simulink model "antiwindup"  (Simulink 4.00)
settings: Solver=ode45  StartTime=0.0  StopTime=2  MaxStep=0.001  RelTol=1e-3
settings Model: LastModifiedBy=Gui

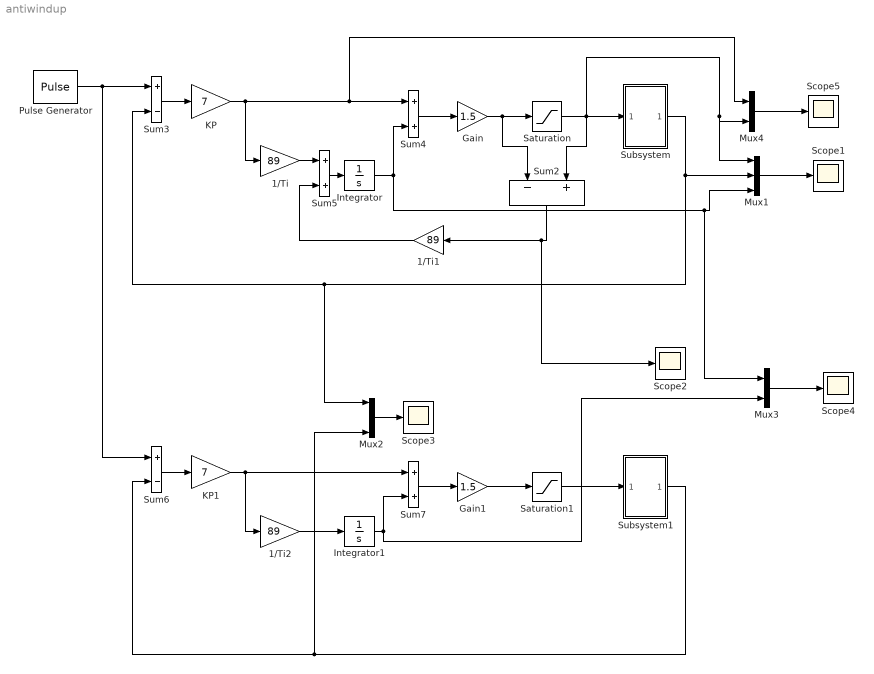
== system antiwindup ==
  1/Ti : Gain  Gain=89  Multiplication=Element-wise(K.*u)  SaturateOnIntegerOverflow=on
  1/Ti1 : Gain  Orientation=left  Gain=89  Multiplication=Element-wise(K.*u)  SaturateOnIntegerOverflow=on
  1/Ti2 : Gain  Gain=89  Multiplication=Element-wise(K.*u)  SaturateOnIntegerOverflow=on
  Gain : Gain  Gain=1.5  Multiplication=Element-wise(K.*u)  SaturateOnIntegerOverflow=on
  Gain1 : Gain  Gain=1.5  Multiplication=Element-wise(K.*u)  SaturateOnIntegerOverflow=on
  Integrator : Integrator  ExternalReset=none  InitialConditionSource=internal  InitialCondition=0  LimitOutput=off  UpperSaturationLimit=inf  LowerSaturationLimit=-inf  ShowSaturationPort=off  ShowStatePort=off  AbsoluteTolerance=auto
  Integrator1 : Integrator  ExternalReset=none  InitialConditionSource=internal  InitialCondition=0  LimitOutput=off  UpperSaturationLimit=inf  LowerSaturationLimit=-inf  ShowSaturationPort=off  ShowStatePort=off  AbsoluteTolerance=auto
  KP : Gain  Gain=7  Multiplication=Element-wise(K.*u)  SaturateOnIntegerOverflow=on
  KP1 : Gain  Gain=7  Multiplication=Element-wise(K.*u)  SaturateOnIntegerOverflow=on
  Mux1 : Mux  Inputs=3
  Mux2 : Mux  Inputs=3
  Mux3 : Mux  Inputs=2
  Mux4 : Mux  Inputs=2
  Pulse Generator : DiscretePulseGenerator  PulseType=Time-based  Amplitude=2  Period=1/5  PulseWidth=50  PhaseDelay=0  SampleTime=1
  Saturation : Saturate  UpperLimit=13.5  LowerLimit=-13.99  LinearizeAsGain=on
  Saturation1 : Saturate  UpperLimit=13.5  LowerLimit=-13.99  LinearizeAsGain=on
  Scope{1..5} (5 alike) : Scope
      Scope1 settings: TimeRange=0.05  YMin=0.2  YMax=1.2  SaveToWorkspace=off  MaxDataPoints=5000
      Scope2 settings: TimeRange=0.05  YMin=-15  YMax=3  SaveToWorkspace=off  SaveName=ScopeData2  MaxDataPoints=5000
      Scope3 settings: TimeRange=0.05  YMin=0.2  YMax=2  SaveToWorkspace=off  SaveName=ScopeData3  MaxDataPoints=5000
      Scope4 settings: TimeRange=0.05  YMin=13.5  YMax=13.5  SaveToWorkspace=off  SaveName=ScopeData4  MaxDataPoints=5000
      Scope5 settings: TimeRange=0.05  YMin=0.2  YMax=1.2  SaveToWorkspace=off  SaveName=ScopeData5  MaxDataPoints=5000
  Subsystem : Subsystem
      settings: RTWFcnNameOpts=Auto  RTWFileNameOpts=Auto
  Subsystem1 : Subsystem
      settings: RTWFcnNameOpts=Auto  RTWFileNameOpts=Auto
  Sum2 : Sum  Orientation=down  Inputs=-+  SaturateOnIntegerOverflow=on
  Sum3 : Sum  Inputs=+-  SaturateOnIntegerOverflow=on
  Sum4 : Sum  Inputs=++  SaturateOnIntegerOverflow=on
  Sum5 : Sum  Inputs=++  SaturateOnIntegerOverflow=on
  Sum6 : Sum  Inputs=+-  SaturateOnIntegerOverflow=on
  Sum7 : Sum  Inputs=++  SaturateOnIntegerOverflow=on
  wires:
  Sum3/1 -> KP/1
  KP/1 -> 1/Ti/1, Sum4/1, Mux4/1
  Gain/1 -> Saturation/1, Sum2/1
  Saturation/1 -> Sum2/2, Mux1/1, Mux4/2, Subsystem/1(In1)
  Sum4/1 -> Gain/1
  1/Ti/1 -> Sum5/1
  Sum5/1 -> Integrator/1
  Integrator/1 -> Sum4/2, Mux1/3, Mux3/1
  Sum2/1 -> 1/Ti1/1, Scope2/1
  1/Ti1/1 -> Sum5/2
  Subsystem/1(Out1) -> Mux1/2, Sum3/2, Mux2/1
  Mux1/1 -> Scope1/1
  Mux2/1 -> Scope3/1
  Sum6/1 -> KP1/1
  KP1/1 -> Sum7/1, 1/Ti2/1
  Gain1/1 -> Saturation1/1
  Saturation1/1 -> Subsystem1/1(In1)
  Sum7/1 -> Gain1/1
  1/Ti2/1 -> Integrator1/1
  Subsystem1/1(Out1) -> Sum6/2, Mux2/3
  Integrator1/1 -> Sum7/2, Mux3/2
  Mux3/1 -> Scope4/1
  Pulse Generator/1 -> Sum3/1, Sum6/1
  Mux4/1 -> Scope5/1

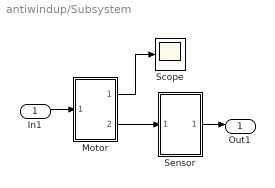
== system antiwindup/Subsystem ==
  In1 : Inport  Port=1  LatchInput=off
  Motor : Subsystem
      settings: RTWFcnNameOpts=Auto  RTWFileNameOpts=Auto
  Scope : Scope
      settings: TimeRange=auto  YMin=-5  YMax=5  SaveToWorkspace=off  SaveName=ScopeData  MaxDataPoints=5000
  Sensor : Subsystem
      settings: RTWFcnNameOpts=Auto  RTWFileNameOpts=Auto
  Out1 : Outport  Port=1
  wires:
  Motor/1(Out1) -> Scope/1
  Motor/2(Out2) -> Sensor/1(In1)
  In1/1 -> Motor/1(In1)
  Sensor/1(Out1) -> Out1/1

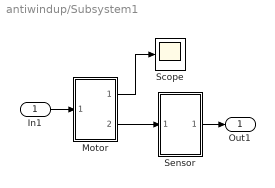
== system antiwindup/Subsystem1 ==
  In1 : Inport  Port=1  LatchInput=off
  Motor : Subsystem
      settings: RTWFcnNameOpts=Auto  RTWFileNameOpts=Auto
  Scope : Scope
      settings: TimeRange=auto  YMin=-5  YMax=5  SaveToWorkspace=off  SaveName=ScopeData  MaxDataPoints=5000
  Sensor : Subsystem
      settings: RTWFcnNameOpts=Auto  RTWFileNameOpts=Auto
  Out1 : Outport  Port=1
  wires:
  Motor/1(Out1) -> Scope/1
  Motor/2(Out2) -> Sensor/1(In1)
  In1/1 -> Motor/1(In1)
  Sensor/1(Out1) -> Out1/1

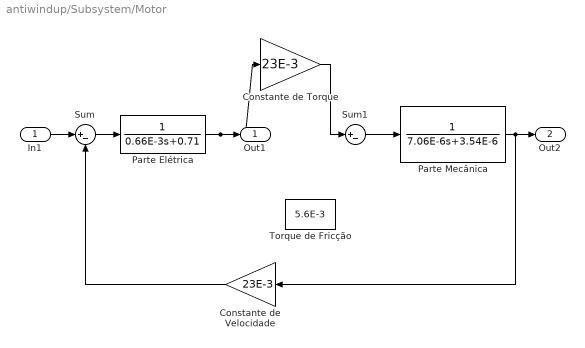
== system antiwindup/Subsystem/Motor ==
  In1 : Inport  Port=1  LatchInput=off
  Constante de Torque : Gain  Gain=23E-3  Multiplication=Element-wise(K.*u)  SaturateOnIntegerOverflow=on
  Constante de Velocidade : Gain  Orientation=left  Gain=23E-3  Multiplication=Element-wise(K.*u)  SaturateOnIntegerOverflow=on
  Parte Elétrica : TransferFcn  Numerator=[1]  Denominator=[0.66E-3 0.71]  AbsoluteTolerance=auto  Realization=auto
  Parte Mecânica : TransferFcn  Numerator=[1]  Denominator=[7.06E-6 3.54E-6]  AbsoluteTolerance=auto  Realization=auto
  Sum : Sum  Inputs=|+-  SaturateOnIntegerOverflow=on
  Sum1 : Sum  Inputs=|+-  SaturateOnIntegerOverflow=on
  Torque de Fricção : Constant  Value=5.6E-3
  Out1 : Outport  Port=1
  Out2 : Outport  Port=2
  wires:
  Sum/1 -> Parte Elétrica/1
  Parte Elétrica/1 -> Constante de Torque/1, Out1/1
  Parte Mecânica/1 -> Constante de Velocidade/1, Out2/1
  Constante de Velocidade/1 -> Sum/2
  Constante de Torque/1 -> Sum1/1
  Sum1/1 -> Parte Mecânica/1
  In1/1 -> Sum/1

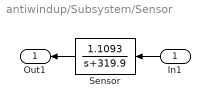
== system antiwindup/Subsystem/Sensor ==
  In1 : Inport  Orientation=left  Port=1  LatchInput=off
  "Sensor " : TransferFcn  Orientation=left  Numerator=[1.1093]  Denominator=[1 319.9]  AbsoluteTolerance=auto  Realization=auto
  Out1 : Outport  Orientation=left  Port=1
  wires:
  "Sensor "/1 -> Out1/1
  In1/1 -> "Sensor "/1

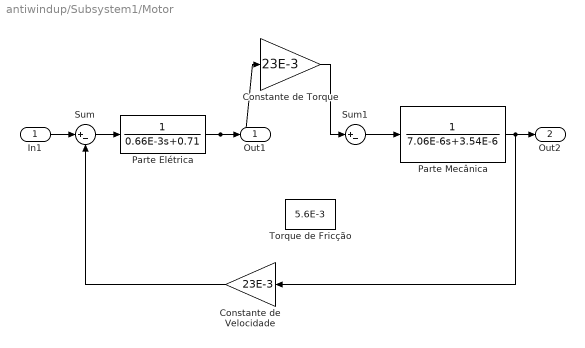
== system antiwindup/Subsystem1/Motor ==
  In1 : Inport  Port=1  LatchInput=off
  Constante de Torque : Gain  Gain=23E-3  Multiplication=Element-wise(K.*u)  SaturateOnIntegerOverflow=on
  Constante de Velocidade : Gain  Orientation=left  Gain=23E-3  Multiplication=Element-wise(K.*u)  SaturateOnIntegerOverflow=on
  Parte Elétrica : TransferFcn  Numerator=[1]  Denominator=[0.66E-3 0.71]  AbsoluteTolerance=auto  Realization=auto
  Parte Mecânica : TransferFcn  Numerator=[1]  Denominator=[7.06E-6 3.54E-6]  AbsoluteTolerance=auto  Realization=auto
  Sum : Sum  Inputs=|+-  SaturateOnIntegerOverflow=on
  Sum1 : Sum  Inputs=|+-  SaturateOnIntegerOverflow=on
  Torque de Fricção : Constant  Value=5.6E-3
  Out1 : Outport  Port=1
  Out2 : Outport  Port=2
  wires:
  Sum/1 -> Parte Elétrica/1
  Parte Elétrica/1 -> Constante de Torque/1, Out1/1
  Parte Mecânica/1 -> Constante de Velocidade/1, Out2/1
  Constante de Velocidade/1 -> Sum/2
  Constante de Torque/1 -> Sum1/1
  Sum1/1 -> Parte Mecânica/1
  In1/1 -> Sum/1

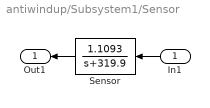
== system antiwindup/Subsystem1/Sensor ==
  In1 : Inport  Orientation=left  Port=1  LatchInput=off
  "Sensor " : TransferFcn  Orientation=left  Numerator=[1.1093]  Denominator=[1 319.9]  AbsoluteTolerance=auto  Realization=auto
  Out1 : Outport  Orientation=left  Port=1
  wires:
  "Sensor "/1 -> Out1/1
  In1/1 -> "Sensor "/1
